simulink model "untitled"  (R2014b)
settings: Solver=ode4  StartTime=0.0  StopTime=5.2  FixedStep=0.001  RelTol=1e-3
libraries: simulink x1
settings Model: Creator=zhoujie  LastModifiedBy=zhoujie

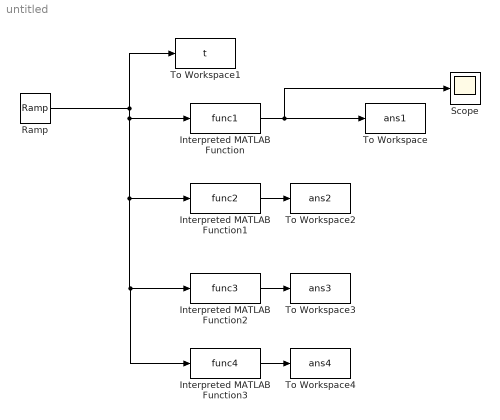
== system untitled ==
  Interpreted MATLAB Function : MATLABFcn  MATLABFcn=func1
  Interpreted MATLAB Function1 : MATLABFcn  MATLABFcn=func2
  Interpreted MATLAB Function2 : MATLABFcn  MATLABFcn=func3
  Interpreted MATLAB Function3 : MATLABFcn  MATLABFcn=func4
  Ramp : simulink/Sources/Ramp  slope=0.1  start=0  X0=0
  Scope : Scope
  To Workspace : ToWorkspace  VariableName=ans1  SaveFormat=Timeseries  SampleTime=-1
  To Workspace1 : ToWorkspace  VariableName=t  SaveFormat=Timeseries  SampleTime=-1
  To Workspace2 : ToWorkspace  VariableName=ans2  SaveFormat=Timeseries  SampleTime=-1
  To Workspace3 : ToWorkspace  VariableName=ans3  SaveFormat=Timeseries  SampleTime=-1
  To Workspace4 : ToWorkspace  VariableName=ans4  SaveFormat=Timeseries  SampleTime=-1
  wires:
  Ramp/1 -> Interpreted MATLAB Function3/1, Interpreted MATLAB Function2/1, Interpreted MATLAB Function1/1, Interpreted MATLAB Function/1, To Workspace1/1
  Interpreted MATLAB Function/1 -> Scope/1, To Workspace/1
  Interpreted MATLAB Function1/1 -> To Workspace2/1
  Interpreted MATLAB Function2/1 -> To Workspace3/1
  Interpreted MATLAB Function3/1 -> To Workspace4/1
